simulink model "outvar"  (Simulink 7.9)
settings: Solver=ode45  SolverMode=SingleTasking  StartTime=0.0  StopTime=10.0  RelTol=1e-3  AbsTol=1e-6
undefined symbols (not defined in the file): den, K, num
settings Model: Creator=Rick  LastModifiedBy=Rick
settings DataIOCC: LimitDataPoints=off
settings OptimizationCC: BlockReduction=off  BooleanDataType=off
settings DebuggingCC: SaveWithParameterizedLinksMsg=none  SignalResolutionControl=TryResolveAllWithWarning  SolverPrmCheckMsg=none  MultiTaskDSMMsg=warning  MultiTaskCondExecSysMsg=none  StrictBusMsg=None
settings HardwareCC: TargetUnknown=on
settings RTWCC: IncludeERTFirstTime=on

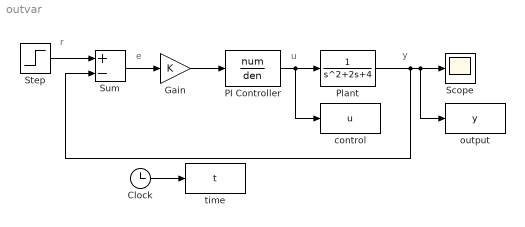
== system outvar ==
  note: y
  note: u
  note: e
  note: r
  Clock : Clock
      settings: DeleteFcn=simclock BlockIsBeingDestroyed  PostSaveFcn=simclock Save
  Gain : Gain  Gain=K  SaturateOnIntegerOverflow=on  OutDataTypeStr=Inherit: Same as input  ParamDataTypeStr=Inherit: Same as input
  PI Controller : TransferFcn  Numerator=num  Denominator=den
  Plant : TransferFcn  Denominator=[1 2 4]
  Scope : Scope
      settings: TickLabels=on
  Step : Step
  Sum : Sum  Inputs=+-  SaturateOnIntegerOverflow=on  InputSameDT=on  OutDataTypeStr=Inherit: Same as first input
  control : ToWorkspace  VariableName=u  SampleTime=-1
  output : ToWorkspace  VariableName=y  SampleTime=-1
  time : ToWorkspace  VariableName=t  SampleTime=-1
  wires:
  PI Controller/1 -> control/1, Plant/1
  Clock/1 -> time/1
  Plant/1 -> output/1, Scope/1, Sum/2
  Gain/1 -> PI Controller/1
  Sum/1 -> Gain/1
  Step/1 -> Sum/1
